simulink model "hw8"  (R2013a)
settings: Solver=ode45  StartTime=0.0  StopTime=35.0  RelTol=1e-3
settings Model: Creator=bazkoale  LastModifiedBy=bazkoale

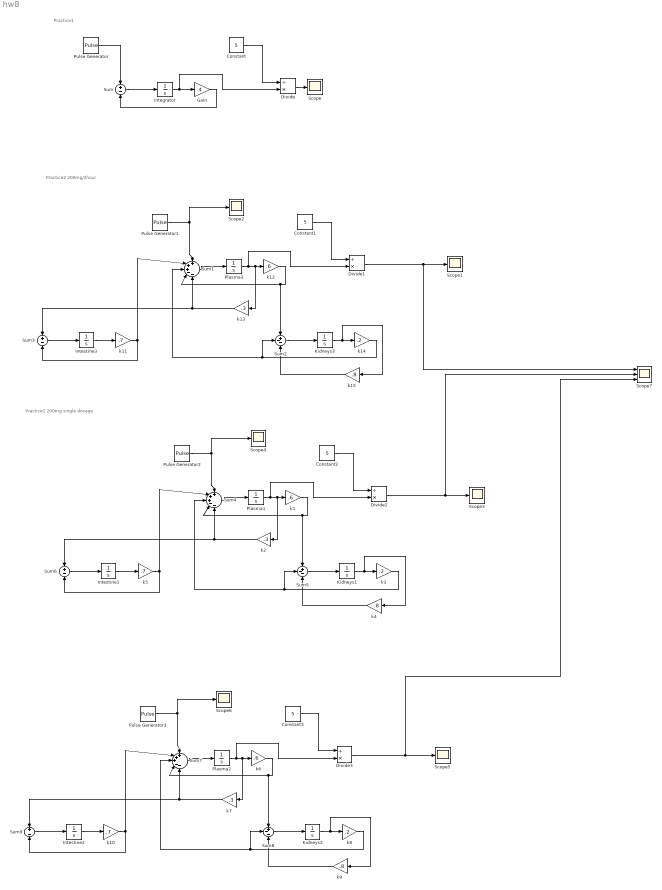
== system hw8 ==
  note: Practice2 200mg/2hour
  note: Practice1
  note: Practice2 200mg single dosage
  Constant{,1..3} (4 alike) : Constant  Value=5
  Divide{,1..3} (4 alike) : Product  Inputs=/*
  Gain : Gain  Gain=.4
  Integrator : Integrator
  Intestine1 : Integrator
  Intestine2 : Integrator
  Intestine3 : Integrator
  Kidneys1 : Integrator
  Kidneys2 : Integrator
  Kidneys3 : Integrator
  Plasma1 : Integrator
  Plasma2 : Integrator  InitialCondition=200
  Plasma3 : Integrator
  Pulse Generator : DiscretePulseGenerator  PulseType=Time based  Amplitude=400/0.07  Period=7
  Pulse Generator1 : DiscretePulseGenerator  PulseType=Time based  Amplitude=200/0.035  Period=35  PulseWidth=0.1
  Pulse Generator2 : DiscretePulseGenerator  PulseType=Time based  Amplitude=200/0.002  PulseWidth=0.1
  Pulse Generator3 : DiscretePulseGenerator  PulseType=Time based  Amplitude=200/0.002  PulseWidth=0.1
  Scope{,1..6} (7 alike) : Scope
      Scope2 settings: SaveName=ScopeData2
      Scope3 settings: SaveName=ScopeData3
      Scope4 settings: SaveName=ScopeData4
      Scope5 settings: SaveName=ScopeData5
      Scope6 settings: SaveName=ScopeData6
  Scope7 : Scope  NumInputPorts=3
      settings: YMin=-5~-5~-5  YMax=5~5~5  SaveName=ScopeData7
  Sum{,3,6,9} (4 alike) : Sum  Inputs=+-
  Sum1 : Sum  Inputs=+++--
  Sum2 : Sum  Inputs=+--
  Sum4 : Sum  Inputs=+++--
  Sum5 : Sum  Inputs=+--
  Sum7 : Sum  Inputs=+++--
  Sum8 : Sum  Inputs=+--
  k1 : Gain  Gain=.6
  k10 : Gain  Gain=.7
  k11 : Gain  Gain=.7
  k12 : Gain  Gain=.6
  k13 : Gain  Gain=.3
  k14 : Gain  Gain=.2
  k15 : Gain  Gain=.8
  k2 : Gain  Gain=.3
  k3 : Gain  Gain=.2
  k4 : Gain  Gain=.8
  k5 : Gain  Gain=.7
  k6 : Gain  Gain=.6
  k7 : Gain  Gain=.3
  k8 : Gain  Gain=.2
  k9 : Gain  Gain=.8
  wires:
  Integrator/1 -> Divide/2, Gain/1
  Gain/1 -> Sum/2
  Sum/1 -> Integrator/1
  Pulse Generator/1 -> Sum/1
  Constant/1 -> Divide/1
  Divide/1 -> Scope/1
  Plasma1/1 -> Divide2/2, k1/1, k2/1
  k1/1 -> Sum5/1, Sum4/4
  Sum4/1 -> Plasma1/1
  Constant2/1 -> Divide2/1
  Divide2/1 -> Scope7/2, Scope3/1
  Kidneys1/1 -> k3/1, k4/1
  k3/1 -> Sum4/3, Sum5/2
  Sum5/1 -> Kidneys1/1
  k4/1 -> Sum5/3
  Intestine1/1 -> k5/1
  k5/1 -> Sum6/2, Sum4/2
  Sum6/1 -> Intestine1/1
  k2/1 -> Sum4/5, Sum6/1
  Pulse Generator2/1 -> Scope4/1, Sum4/1
  Plasma2/1 -> k7/1, k6/1, Divide3/2
  k6/1 -> Sum7/4, Sum8/1
  Sum7/1 -> Plasma2/1
  Constant3/1 -> Divide3/1
  Divide3/1 -> Scope7/3, Scope5/1
  Kidneys2/1 -> k9/1, k8/1
  k8/1 -> Sum8/2, Sum7/3
  Sum8/1 -> Kidneys2/1
  k9/1 -> Sum8/3
  Intestine2/1 -> k10/1
  k10/1 -> Sum7/2, Sum9/2
  Sum9/1 -> Intestine2/1
  k7/1 -> Sum9/1, Sum7/5
  Pulse Generator3/1 -> Sum7/1, Scope6/1
  Plasma3/1 -> Divide1/2, k12/1, k13/1
  k12/1 -> Sum2/1, Sum1/4
  Sum1/1 -> Plasma3/1
  Constant1/1 -> Divide1/1
  Divide1/1 -> Scope7/1, Scope1/1
  Kidneys3/1 -> k14/1, k15/1
  k14/1 -> Sum1/3, Sum2/2
  Sum2/1 -> Kidneys3/1
  k15/1 -> Sum2/3
  Intestine3/1 -> k11/1
  k11/1 -> Sum3/2, Sum1/2
  Sum3/1 -> Intestine3/1
  k13/1 -> Sum1/5, Sum3/1
  Pulse Generator1/1 -> Scope2/1, Sum1/1
